simulink model "stream_data"  (R2018b)
settings: Solver=VariableStepAuto  StartTime=0.0  StopTime=10.0  RelTol=1e-3
settings Model: Creator=diyar  LastModifiedBy=diyar

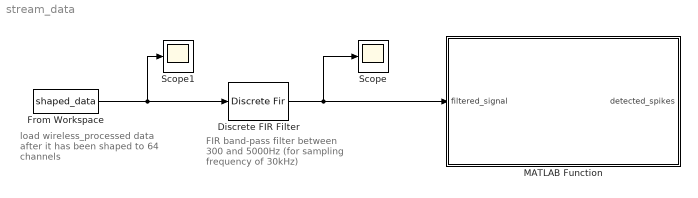
== system stream_data ==
  note: FIR band-pass filter between 300 and 5000Hz (for sampling frequency of 30kHz)
  note: load wireless_processed data after it has been shaped to 64 channels
  Discrete FIR Filter : DiscreteFir  Coefficients="[-0.00256460955632912\t-0.00122763189978458\t0.000415589924103434\t0.000235493840983018\t-0.00460315453054656\t-0.0127730960261749\t-0.0161479251552066\t-0.00701917991322031\t0.00907070223480388\t0.0114671711523351\t-0.0163341202375131\t-0.0606478474288596\t-0.0750999922056138\t-0.0152334366069452\t0.115089684764604\t0.251213077711346\t0.309337809429954\t0.251213077711346\t0.115089684764604\t-0.0152334366069452\t-0.0750999922056138\t-0.0606478474288596\t-0.0163341202375131\t0.0114671711523351\t0.00907070223480388\t-0.00701917991322031\t-0.0161479251552066\t-0.0127730960261749\t-0.00460315453054656\t0.000235493840983018\t0.000415589924103434\t-0.00122763189978458\t-0.00256460955632912]"  InputProcessing=Columns as channels (frame based)
  From Workspace : FromWorkspace  VariableName=shaped_data  OutDataTypeStr=double  OutputAfterFinalValue=Setting to zero
  MATLAB Function : MATLAB Function  TreatAsAtomicUnit=on
  Scope : Scope
  Scope1 : Scope
  wires:
  From Workspace/1 -> Scope1/1, Discrete FIR Filter/1
  Discrete FIR Filter/1 -> MATLAB Function/1(filtered_signal), Scope/1

== matlab function stream_data/MATLAB Function ==
  data: filtered_signal input; detected_spikes output
function detected_spikes = spike_detect(filtered_signal)

detected_spikes = filtered_signal;
